simulink model "IIR_Filter_PIL_Int32"  (Simulink 8.6)
settings: Solver=FixedStepDiscrete  StartTime=0.0  StopTime=1  FixedStep=0.001  RelTol=1e-3
model workspace (MAT data in the model file):
  dataint = Simulink.Signal
  dataint.DataType = 'int32'
  dataint.Units = 'auto'
  dataint.Dimensions = -1
  dataint.DimensionsMode = 'auto'
  dataint.Complexity = 'real'
  dataint.SampleTime = -1
  dataint.SamplingMode = 'auto'
  dataint.InitialValue = '0'
PreLoadFcn:
  | run iir_startup;
libraries: simulink x1
settings Model: DataTypeOverrideAppliesTo=Floating-point  Creator=obas  LastModifiedBy=reynaudp
settings DataIOCC: ExternalInput=[t, testdata]  FinalStateName=xFinal_PIL  LimitDataPoints=off  LoadExternalInput=on  SignalLogging=off  StateSaveName=xout_PIL  TimeSaveName=tout_PIL  OutputSaveName=yout_PIL  SignalLoggingName=logsOut_PIL
settings OptimizationCC: DefaultParameterBehavior=Inlined  ZeroExternalMemoryAtStartup=off  ZeroInternalMemoryAtStartup=off  OptimizeModelRefInitCode=on  LifeSpan=1
settings DebuggingCC: SaveWithParameterizedLinksMsg=none  CheckExecutionContextPreStartOutputMsg=on  CheckExecutionContextRuntimeOutputMsg=on  SignalResolutionControl=TryResolveAllWithWarning  MultiTaskDSMMsg=warning  MultiTaskCondExecSysMsg=none  ParameterPrecisionLossMsg=none  FcnCallInpInsideContextMsg=UseLocalSettings  StrictBusMsg=ErrorOnBusTreatedAsVector
settings HardwareCC: ProdLargestAtomicInteger=Integer  ProdLargestAtomicFloat=Float  ProdIntDivRoundTo=Zero  ProdEndianess=LittleEndian  ProdHWDeviceType=STMicroelectronics->STM32 32-bit Cortex-M
settings SFSimCC: SimUserSources=stm32f4xx_rcc
settings RTWCC: SystemTargetFile=stm32.tlc  TemplateMakefile=stm32.tmf  Description=stm32 (Embedded Target)  GenerateReport=on  IncludeHyperlinkInReport=on  LaunchReport=on  CodeExecutionProfiling=on  CodeProfilingInstrumentation=on  GenerateCodeReplacementReport=on
settings CodeAppCC: IgnoreCustomStorageClasses=off  MaxIdLength=64  CustomSymbolStrType=$N$R$M  InternalIdentifier=Classic
settings STFCustomTargetCC: CodeReplacementLibrary=ARM CMSIS SIN COS  ParMdlRefBuildCompliant=on  IncludeMdlTerminateFcn=off  CombineOutputUpdateFcns=on  ERTCustomFileBanners=on  SupportContinuousTime=off  SupportNonInlinedSFcns=off  MATLABClassNameForMDSCustomization=Simulink.SoftwareTarget.ERTCustomization  GRTInterface=off  SystemTargetFile=stm32.tlc
settings ERTTargetCC: CodeReplacementLibrary=ARM CMSIS SIN COS  MultiwordLength=2048  CompOptLevelCompliant=off  ConcurrentExecutionCompliant=off  IncludeMdlTerminateFcn=off  ERTFirstTimeCompliant=off  ModelStepFunctionPrototypeControlCompliant=off  CPPClassGenCompliant=off  UseToolchainInfoCompliant=off  InlinedParameterPlacement=NonHierarchical  ERTSrcFileBannerTemplate=sourceFileTemplate.cgt  ERTHdrFileBannerTemplate=sourceFileTemplate.cgt  ERTDataSrcFileTemplate=sourceFileTemplate.cgt  ERTDataHdrFileTemplate=sourceFileTemplate.cgt  ERTCustomFileTemplate=customRoutineProcess.tlc  ConvertIfToSwitch=off  SuppressUnreachableDefaultCases=off
settings CustomProperty: Value=on
settings ConfigComp: CovSFcnEnable=off

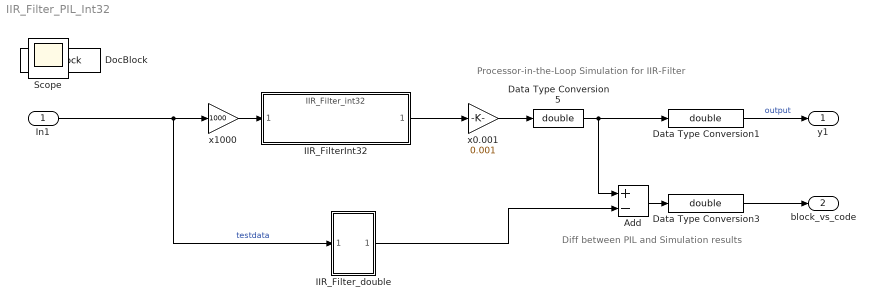
== system IIR_Filter_PIL_Int32 ==
  note: Diff between PIL and Simulation results
  note: Processor-in-the-Loop Simulation for IIR-Filter
  In1 : Inport  OutDataTypeStr=double
  Add : Sum  Inputs=+-
  Data Type Conversion1 : DataTypeConversion  OutDataTypeStr=double  SaturateOnIntegerOverflow=on  RndMeth=Zero
  Data Type Conversion3 : DataTypeConversion  OutDataTypeStr=double  SaturateOnIntegerOverflow=on  RndMeth=Zero
  Data Type Conversion5 : DataTypeConversion  OutDataTypeStr=double  SaturateOnIntegerOverflow=on  RndMeth=Zero
  DocBlock : simulink/Model-Wide Utilities/DocBlock  DocumentType=Text
      content=|
      | The model contains a 1st-order IIR filter of the following form:
      |
      |     y(n) = a1*y(n-1) + b0*u(n)
      |
      | Using the model pre-load function callback:
      |
      |     a1 = 0.9
      |     b0 = 0.1
      |
      | The filter is sampled at 1000Hz.
      |
      | Modified from iir_filter.mdl to enable ERT code generation.
  IIR_FilterInt32 : ModelReference  ModelNameDialog=IIR_Filter_int32  SimulationMode=Processor-in-the-loop (PIL)  ModelReferenceVersion=1.103  CopyOfModelName=IIR_Filter_int32
  IIR_Filter_double : Subsystem
  x0.001 : Gain  Gain=0.001
  x1000 : Gain  Gain=1000  ParamDataTypeStr=uint32  OutMin=-2147483647-1  OutMax=2147483647  OutDataTypeStr=int32
  y1 : Outport
  block_vs_code : Outport  Port=2
  Scope : Scope
  wires:
  In1/1 -> x1000/1, IIR_Filter_double/1(Input)  "testdata"
  Data Type Conversion1/1 -> y1/1  "output"
  Data Type Conversion3/1 -> block_vs_code/1
  Add/1 -> Data Type Conversion3/1
  Data Type Conversion5/1 -> Add/1, Data Type Conversion1/1
  x0.001/1 -> Data Type Conversion5/1
  IIR_Filter_double/1(Output) -> Add/2
  x1000/1 -> IIR_FilterInt32/1
  IIR_FilterInt32/1 -> x0.001/1

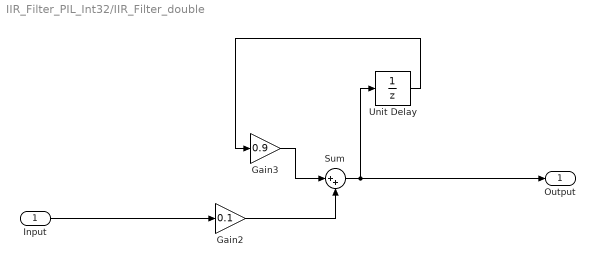
== system IIR_Filter_PIL_Int32/IIR_Filter_double ==
  Input : Inport  LockScale=on
  Gain2 : Gain  Gain=0.1
  Gain3 : Gain  Gain=0.9  OutDataTypeStr=Inherit: Inherit via back propagation
  Sum : Sum  Inputs=|++  OutDataTypeStr=double
  Unit Delay : UnitDelay  SampleTime=-1
  Output : Outport
  wires:
  Gain2/1 -> Sum/2
  Sum/1 -> Unit Delay/1, Output/1
  Gain3/1 -> Sum/1
  Unit Delay/1 -> Gain3/1
  Input/1 -> Gain2/1
